simulink model "StateflowBlock"  (R2024a)
settings: Solver=FixedStepDiscrete  StartTime=0.0  StopTime=Inf  FixedStep=0.1  RelTol=1e-3
settings Model: TunableVars=kp,PWMsl_l,PWMsl_r,PWMsr_l,PWMsr_r  TunableVarsStorageClass=Auto,Auto,Auto,Auto,Auto  TunableVarsTypeQualifier=,,,,  Creator=omars  LastModifiedBy=lukas
settings DataIOCC: ReturnWorkspaceOutputs=off
settings OptimizationCC: EnhancedBackFolding=on  PassReuseOutputArgsAs=Individual arguments  ZeroExternalMemoryAtStartup=off  ZeroInternalMemoryAtStartup=off  OptimizeBlockOrder=speed  DifferentSizesBufferReuse=on  OptimizationCustomize=off  EfficientTunableParamExpr=on
settings DebuggingCC: ParameterTunabilityLossMsg=error
settings SFSimCC: MATLABDynamicMemAlloc=off
settings RTWCC: Description=Embedded Coder  SystemTargetFile=ert.tlc  GenCodeOnly=on  TemplateMakefile=ert_default_tmf  GPUComputeCapability=3.5
settings CodeAppCC: ForceParamTrailComments=on  IgnoreCustomStorageClasses=off  OperatorAnnotations=on  SimulinkDataObjDesc=on  SFDataObjDesc=on  InsertBlockDesc=on
settings ERTTargetCC: TargetLangStandard=C99 (ISO)  ERTCustomFileTemplate=example_file_process.tlc

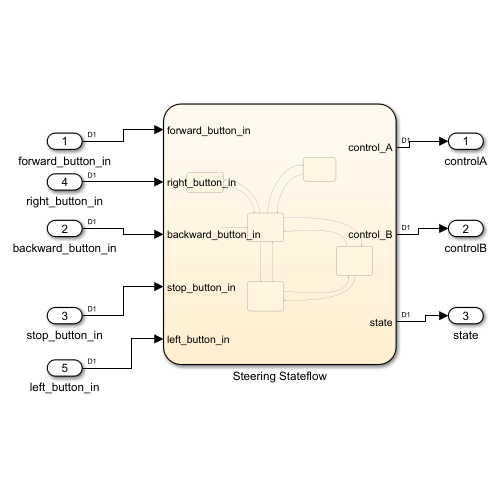
[thumbnail: Simulink's stored preview of the top-level diagram]
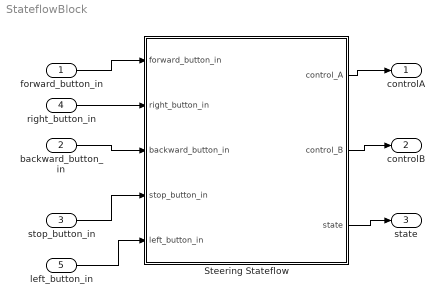
== system StateflowBlock ==
  forward_button_in : Inport
  backward_button_in : Inport  Port=2
  stop_button_in : Inport  Port=3
  right_button_in : Inport  Port=4
  left_button_in : Inport  Port=5
  Steering Stateflow : Stateflow chart  TreatAsAtomicUnit=on
  controlA : Outport
  controlB : Outport  Port=2
  state : Outport  Port=3
  wires:
  stop_button_in/1 -> Steering Stateflow/4(stop_button_in)
  Steering Stateflow/2(control_B) -> controlB/1
  Steering Stateflow/3(state) -> state/1
  Steering Stateflow/1(control_A) -> controlA/1
  backward_button_in/1 -> Steering Stateflow/3(backward_button_in)
  forward_button_in/1 -> Steering Stateflow/1(forward_button_in)
  right_button_in/1 -> Steering Stateflow/2(right_button_in)
  left_button_in/1 -> Steering Stateflow/5(left_button_in)

== stateflow chart StateflowBlock/Steering Stateflow ==
  settings: updateMethod=DISCRETE  sampleTime=0.1
  state Turn_Right
    control_A = 0.5;
    control_B = 0.5;
    state = 4;
  state Idle
    control_A = 0;
    control_B = 0;
    state = 0;
  state Backward
    control_A = 0.5;
    control_B = -0.5;
    state = 2;
  state Forward
    control_A = -0.5;
    control_B = 0.5;
    state = 1;
  state Turn_Left
    control_A = -0.5;
    control_B = -0.5;
    state = 3;
  Forward -> Turn_Right [order 4] : [right_button_in > 0]
  Turn_Right -> Forward [order 3] : [forward_button_in > 0]
  Idle -> Turn_Right [order 3] : [right_button_in > 0]
  Turn_Right -> Idle [order 1] : [stop_button_in > 0]
  Backward -> Turn_Right [order 3] : [right_button_in > 0]
  Turn_Right -> Backward [order 2] : [backward_button_in > 0]
  Idle -> Backward [order 2] : [backward_button_in > 0]
  (default) -> Idle
  Backward -> Idle [order 2] : [stop_button_in > 0]
  Idle -> Forward [order 1] : [forward_button_in> 0]
  Idle -> Turn_Left [order 4] : [left_button_in > 0]
  Forward -> Idle [order 1] : [stop_button_in > 0]
  Turn_Left -> Idle [order 1] : [stop_button_in > 0]
  Forward -> Backward [order 2] : [backward_button_in > 0]
  Backward -> Forward [order 1] : [forward_button_in > 0]
  Turn_Left -> Backward [order 3] : [backward_button_in > 0]
  Backward -> Turn_Left [order 4] : [left_button_in > 0]
  Turn_Left -> Forward [order 2] : [forward_button_in > 0]
  Forward -> Turn_Left [order 3] : [left_button_in > 0]
  data: forward_button_in input boolean; right_button_in input; backward_button_in input boolean; control_A output double; control_B output double; stop_button_in input boolean =500; state output; left_button_in input
